simulink model "qftdm1_sim"  (Simulink 5.0)
settings: Solver=ode45  StartTime=0.0  StopTime=10  RelTol=1e-3
values from neighbouring files (symbols this model uses):
  k = 30    [chap8_5ctrl.m]    (also in chap8_6ctrl.m = 2; qft_int.m = 1; qftdm1_int.m = 379; qftdm1_plant.m = 1)
  p1 = 123.5+213.9i    [qftdm1_int.m]    (also in qftdm2_int.m = 42.81)
  p2 = P(1,2)    [chap8_1ctrl.m]    (also in chap8_2ctrl.m; qftdm1_int.m = 123.5-213.9i; qftdm2_int.m = 743+669.3i)
  z1 = 42    [qftdm1_int.m]    (also in qftdm2_int.m = 1.1)
settings Model: LastModifiedBy=Administrator  ExtModeTrigMode=oneshot  ExtModeArmWhenConnect=off  LimitDataPoints=off  BooleanDataType=off

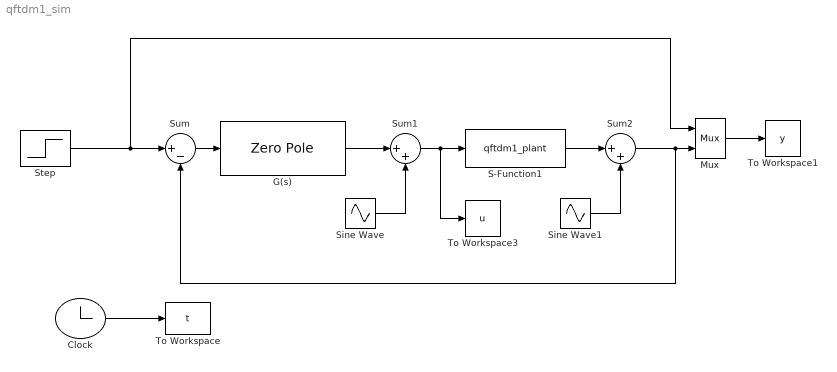
== system qftdm1_sim ==
  Clock : Clock
  G(s) : ZeroPole  Zeros=[-z1]  Poles=[-p1 -p2]  Gain=[k*(p1*p2)/z1]
  Mux : Mux  Inputs=2
  S-Function1 : S-Function  FunctionName=qftdm1_plant
  Sine Wave : Sin  Amplitude=3  SampleTime=0
  Sine Wave1 : Sin  Amplitude=0.02  Frequency=10  SampleTime=0
  Step : Step  Time=0  SampleTime=0
  Sum : Sum  Inputs=|+-  SaturateOnIntegerOverflow=on  InputSameDT=on
  Sum1 : Sum  Inputs=|++  SaturateOnIntegerOverflow=on  InputSameDT=on
  Sum2 : Sum  Inputs=|++  SaturateOnIntegerOverflow=on  InputSameDT=on
  To Workspace : ToWorkspace  VariableName=t  SampleTime=-1  SaveFormat=Array
  To Workspace1 : ToWorkspace  VariableName=y  SampleTime=-1  SaveFormat=Array
  To Workspace3 : ToWorkspace  VariableName=u  SampleTime=-1  SaveFormat=Array
  wires:
  Clock/1 -> To Workspace/1
  Sum/1 -> G(s)/1
  Step/1 -> Sum/1, Mux/1
  Mux/1 -> To Workspace1/1
  S-Function1/1 -> Sum2/1
  Sine Wave1/1 -> Sum2/2
  Sum2/1 -> Mux/2, Sum/2
  Sine Wave/1 -> Sum1/2
  G(s)/1 -> Sum1/1
  Sum1/1 -> S-Function1/1, To Workspace3/1
